simulink model "Fahrrad"  (Simulink 7.6)
settings: Solver=ode45  StartTime=0.0  StopTime=10.0  RelTol=1e-3
undefined symbols (not defined in the file): i, Kd, Ki, Kp, tau
settings Model: Creator=Markus  LastModifiedBy=Markus

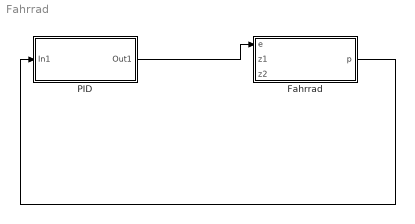
== system Fahrrad ==
  Fahrrad : Subsystem
  PID : Subsystem
  wires:
  PID/1(Out1) -> Fahrrad/1(e)
  Fahrrad/1(p) -> PID/1(In1)

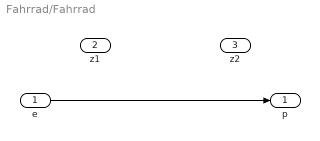
== system Fahrrad/Fahrrad ==
  e : Inport
  z1 : Inport  Port=2
  z2 : Inport  Port=3
  p : Outport
  wires:
  e/1 -> p/1

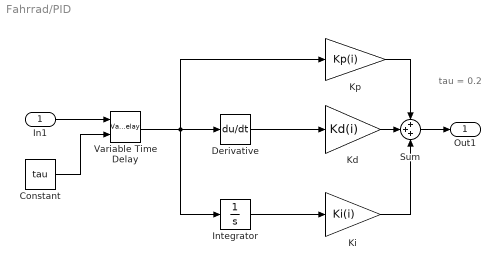
== system Fahrrad/PID ==
  note: tau = 0.2
  In1 : Inport
  Constant : Constant  Value=tau
  Derivative : Derivative
  Integrator : Integrator
  Kd : Gain  Gain=Kd(i)
  Ki : Gain  Gain=Ki(i)
  Kp : Gain  Gain=Kp(i)
  Sum : Sum  Inputs=+++
  Variable Time Delay : VariableTransportDelay  MaximumDelay=10
  Out1 : Outport
  wires:
  Kp/1 -> Sum/1
  Sum/1 -> Out1/1
  Variable Time Delay/1 -> Derivative/1, Kp/1, Integrator/1
  In1/1 -> Variable Time Delay/1
  Constant/1 -> Variable Time Delay/2
  Integrator/1 -> Ki/1
  Derivative/1 -> Kd/1
  Kd/1 -> Sum/2
  Ki/1 -> Sum/3
